simulink model "rho_2_exp"  (R2014a)
settings: Solver=ode45  StartTime=0.0  StopTime=20  RelTol=1e-3
undefined symbols (not defined in the file): A, alpha, B, C, D, k1, k2, mu, nu, sigma
settings Model: Creator=Олег  LastModifiedBy=пользователь

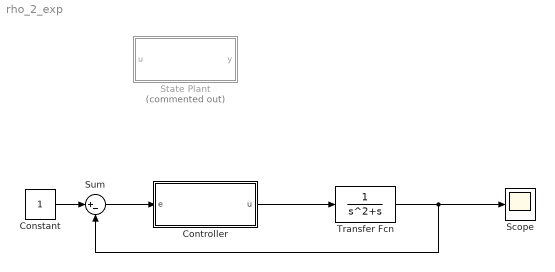
== system rho_2_exp ==
  Constant : Constant
  Controller : Subsystem
  Scope : Scope
      settings: TimeRange=20  YMin=0  YMax=6500
  State Plant : Subsystem  Commented=on
  Sum : Sum  Inputs=|+-
  Transfer Fcn : TransferFcn  Denominator=[1 1 0]
  wires:
  Constant/1 -> Sum/1
  Transfer Fcn/1 -> Sum/2, Scope/1
  Sum/1 -> Controller/1(e)
  Controller/1(u) -> Transfer Fcn/1

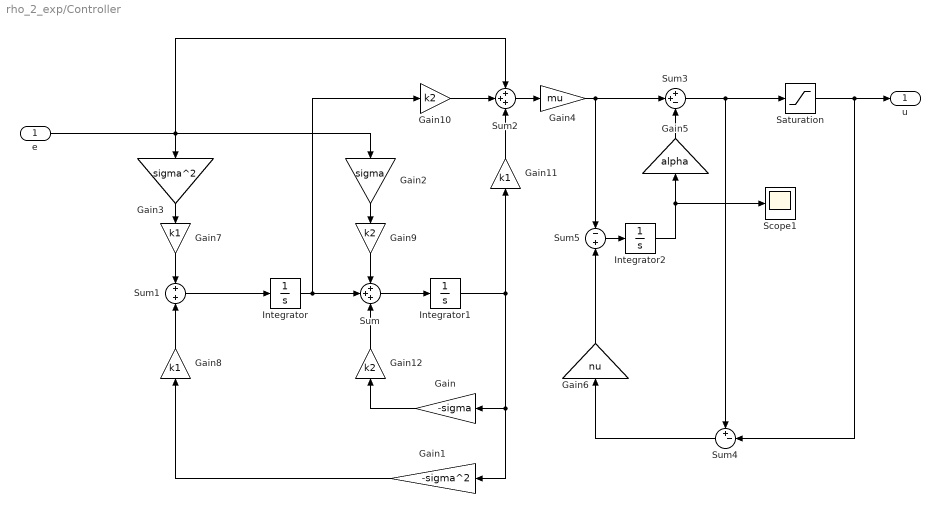
== system rho_2_exp/Controller ==
  e : Inport
  Gain : Gain  Gain=-sigma
  Gain1 : Gain  Gain=-sigma^2
  Gain10 : Gain  Gain=k2
  Gain11 : Gain  Gain=k1
  Gain12 : Gain  Gain=k2
  Gain2 : Gain  Gain=sigma
  Gain3 : Gain  Gain=sigma^2
  Gain4 : Gain  Gain=mu
  Gain5 : Gain  Gain=alpha
  Gain6 : Gain  Gain=nu
  Gain7 : Gain  Gain=k1
  Gain8 : Gain  Gain=k1
  Gain9 : Gain  Gain=k2
  Integrator : Integrator
  Integrator1 : Integrator
  Integrator2 : Integrator
  Saturation : Saturate  UpperLimit=5  LowerLimit=-5
  Scope1 : Scope
      settings: SaveName=ScopeData2
  Sum : Sum  Inputs=+++
  Sum1 : Sum
  Sum2 : Sum  Inputs=+++
  Sum3 : Sum  Inputs=++-
  Sum4 : Sum  Inputs=+-|
  Sum5 : Sum  Inputs=-+
  u : Outport
  wires:
  Sum1/1 -> Integrator/1
  Integrator/1 -> Gain10/1, Sum/2
  Sum/1 -> Integrator1/1
  Integrator1/1 -> Gain1/1, Gain/1, Gain11/1
  Gain/1 -> Gain12/1
  Gain1/1 -> Gain8/1
  Gain2/1 -> Gain9/1
  Gain3/1 -> Gain7/1
  Sum2/1 -> Gain4/1
  Sum3/1 -> Saturation/1, Sum4/1
  Sum5/1 -> Integrator2/1
  Integrator2/1 -> Gain5/1, Scope1/1
  Sum4/1 -> Gain6/1
  Gain4/1 -> Sum5/1, Sum3/2
  e/1 -> Gain3/1, Gain2/1, Sum2/1
  Gain5/1 -> Sum3/3
  Gain6/1 -> Sum5/2
  Saturation/1 -> Sum4/2, u/1
  Gain7/1 -> Sum1/1
  Gain9/1 -> Sum/1
  Gain8/1 -> Sum1/2
  Gain10/1 -> Sum2/2
  Gain11/1 -> Sum2/3
  Gain12/1 -> Sum/3

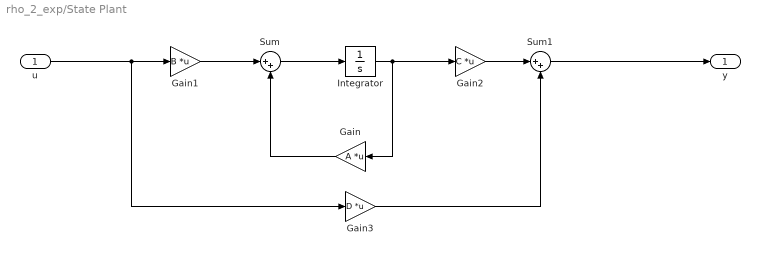
== system rho_2_exp/State Plant ==
  u : Inport
  Gain : Gain  Gain=A  Multiplication=Matrix(K*u)
  Gain1 : Gain  Gain=B  Multiplication=Matrix(K*u)
  Gain2 : Gain  Gain=C  Multiplication=Matrix(K*u)
  Gain3 : Gain  Gain=D  Multiplication=Matrix(K*u)
  Integrator : Integrator  InitialCondition=[0;0]
  Sum : Sum  Inputs=|++
  Sum1 : Sum  Inputs=|++
  y : Outport
  wires:
  Integrator/1 -> Gain2/1, Gain/1
  Sum/1 -> Integrator/1
  Gain/1 -> Sum/2
  Gain1/1 -> Sum/1
  u/1 -> Gain3/1, Gain1/1
  Gain2/1 -> Sum1/1
  Sum1/1 -> y/1
  Gain3/1 -> Sum1/2
